simulink model "TomaDatosOrden1MismaEnt"  (R2018b)
settings: Solver=VariableStepAuto  StartTime=0.0  StopTime=120  RelTol=1e-3
values from neighbouring files (symbols this model uses):
  Input = 1    [DatosPrimerOrdenK10Input1.mat]    (also in DatosPrimerOrdenK1Input1.mat; DatosPrimerOrdenK5Input1.mat)
  K = 10    [DatosPrimerOrdenK10Input1.mat]    (also in DatosPrimerOrdenK1Input1.mat = 1; DatosPrimerOrdenK5Input1.mat = 5)
settings Model: Creator=root  LastModifiedBy=root
settings SFSimCC: SimUseLocalCustomCode=off
settings RTWCC: RTWUseLocalCustomCode=off
settings CodeAppCC: StateflowObjectComments=on

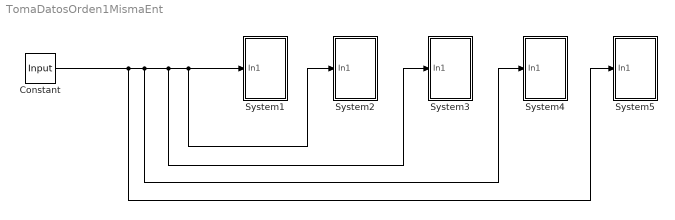
== system TomaDatosOrden1MismaEnt ==
  Constant : Constant  Value=Input
  System1 : Subsystem
  System2 : Subsystem
  System3 : Subsystem
  System4 : Subsystem
  System5 : Subsystem
  wires:
  Constant/1 -> System5/1(In1), System4/1(In1), System3/1(In1), System2/1(In1), System1/1(In1)

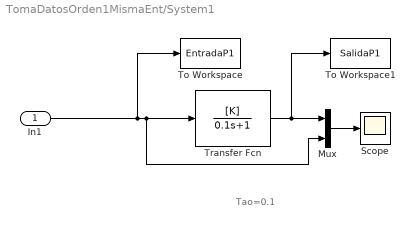
== system TomaDatosOrden1MismaEnt/System1 ==
  note: Tao=0.1
  In1 : Inport
  Mux : Mux  Inputs=2
  Scope : Scope
  To Workspace : ToWorkspace  VariableName=EntradaP1  SampleTime=0.01
  To Workspace1 : ToWorkspace  VariableName=SalidaP1  SampleTime=0.01
  Transfer Fcn : TransferFcn  Numerator=[K]  Denominator=[0.1 1]
  wires:
  Mux/1 -> Scope/1
  In1/1 -> To Workspace/1, Mux/2, Transfer Fcn/1
  Transfer Fcn/1 -> To Workspace1/1, Mux/1

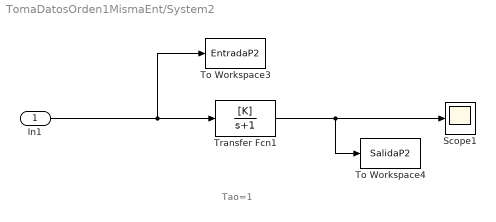
== system TomaDatosOrden1MismaEnt/System2 ==
  note: Tao=1
  In1 : Inport
  Scope1 : Scope
  To Workspace3 : ToWorkspace  VariableName=EntradaP2  SampleTime=0.01
  To Workspace4 : ToWorkspace  VariableName=SalidaP2  SampleTime=0.01
  Transfer Fcn1 : TransferFcn  Numerator=[K]  Denominator=[1 1]
  wires:
  Transfer Fcn1/1 -> To Workspace4/1, Scope1/1
  In1/1 -> To Workspace3/1, Transfer Fcn1/1

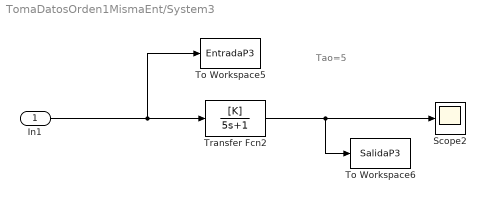
== system TomaDatosOrden1MismaEnt/System3 ==
  note: Tao=5
  In1 : Inport
  Scope2 : Scope
  To Workspace5 : ToWorkspace  VariableName=EntradaP3  SampleTime=0.01
  To Workspace6 : ToWorkspace  VariableName=SalidaP3  SampleTime=0.01
  Transfer Fcn2 : TransferFcn  Numerator=[K]  Denominator=[5 1]
  wires:
  Transfer Fcn2/1 -> To Workspace6/1, Scope2/1
  In1/1 -> To Workspace5/1, Transfer Fcn2/1

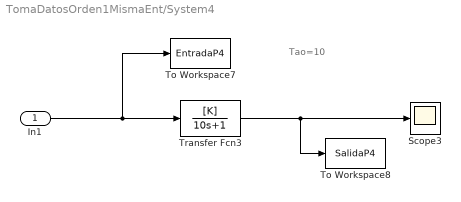
== system TomaDatosOrden1MismaEnt/System4 ==
  note: Tao=10
  In1 : Inport
  Scope3 : Scope
  To Workspace7 : ToWorkspace  VariableName=EntradaP4  SampleTime=0.01
  To Workspace8 : ToWorkspace  VariableName=SalidaP4  SampleTime=0.01
  Transfer Fcn3 : TransferFcn  Numerator=[K]  Denominator=[10 1]
  wires:
  Transfer Fcn3/1 -> To Workspace8/1, Scope3/1
  In1/1 -> To Workspace7/1, Transfer Fcn3/1

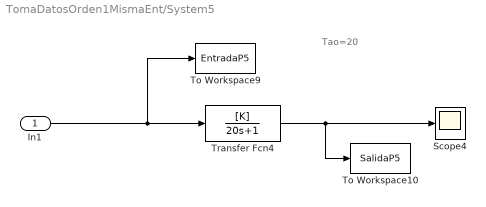
== system TomaDatosOrden1MismaEnt/System5 ==
  note: Tao=20
  In1 : Inport
  Scope4 : Scope
  To Workspace10 : ToWorkspace  VariableName=SalidaP5  SampleTime=0.01
  To Workspace9 : ToWorkspace  VariableName=EntradaP5  SampleTime=0.01
  Transfer Fcn4 : TransferFcn  Numerator=[K]  Denominator=[20 1]
  wires:
  Transfer Fcn4/1 -> To Workspace10/1, Scope4/1
  In1/1 -> To Workspace9/1, Transfer Fcn4/1
